simulink model "aa"  (R2025b)
settings: Solver=FixedStepAuto  StartTime=0.0  StopTime=10.0  RelTol=1e-3
libraries: androiduilib x2, dspxfrm3 x2, androidaudiovideolib x1, commchan3 x1, androidcommunicationlib x1
settings Model: Creator=chinm  LastModifiedBy=Windows
settings OptimizationCC: DefaultParameterBehavior=Inlined  EnhancedBackFolding=on  PassReuseOutputArgsAs=Individual arguments  ZeroExternalMemoryAtStartup=off  ZeroInternalMemoryAtStartup=off  MaxStackSize=64  OptimizeBlockOrder=speed  DifferentSizesBufferReuse=on  OptimizationCustomize=off  EfficientTunableParamExpr=on
settings DebuggingCC: ParameterTunabilityLossMsg=error
settings HardwareCC: ProdBitPerPointer=32.0  ProdBitPerSizeT=32.0  ProdBitPerPtrDiffT=32.0  ProdLargestAtomicInteger=Long  ProdLargestAtomicFloat=Double  ProdWordSize=32.0  ProdHWDeviceType=ARM Compatible->ARM Cortex-A (32-bit)
settings SFSimCC: MATLABDynamicMemAlloc=off
settings RTWCC: SystemTargetFile=ert.tlc  HardwareBoard=Android Device  TLCOptions="-aInlineSetEventsForThisBaseRateFcn=TLC_FALSE -aSuppressMultiTaskScheduler=TLC_FALSE  -aRateBasedStepFcn=0"  TemplateMakefile=ert_default_tmf  RTWVerbose=off  Toolchain=Android SDK/NDK Tools  GPUComputeCapability=3.5  Description=Embedded Coder
settings CodeAppCC: ForceParamTrailComments=on  IgnoreCustomStorageClasses=off  OperatorAnnotations=on  SimulinkDataObjDesc=on  SFDataObjDesc=on  InsertBlockDesc=on

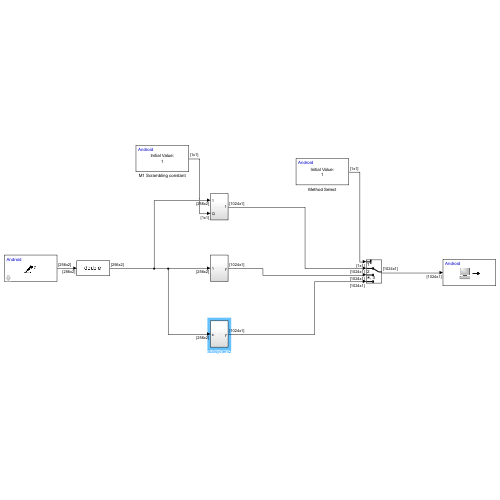
[thumbnail: Simulink's stored preview of the top-level diagram]
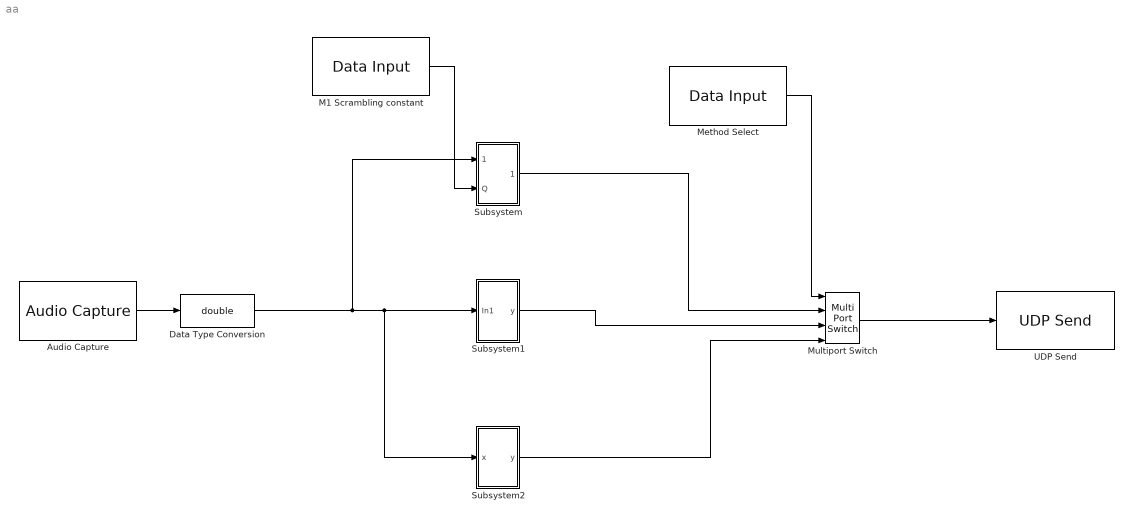
== system aa ==
  Audio Capture : androidaudiovideolib/Audio Capture  SampleFreq=8000  FrameSize=256  SampleTime=0.032  SimulateUsing=Code generation  DeviceStr=0  QueueDuration=0  BlockPlatform=Android  AudioSamplingFreq=44100
  Data Type Conversion : DataTypeConversion  OutDataTypeStr=double  SaturateOnIntegerOverflow=off  RndMeth=Floor
  M1 Scrambling constant : androiduilib/Data Input  isCharVector=off  Value=1.0  CharVector=Hello World  OutputDataType=int8  maxCharVectorSize=100  DataInputId=aa/M1_Scrambling_constant  SampleTime=1
  Method Select : androiduilib/Data Input  isCharVector=off  Value=1  CharVector=Hello World  OutputDataType=int8  maxCharVectorSize=100  DataInputId=aa/Method_Select  SampleTime=1
  Multiport Switch : MultiPortSwitch  DataPortOrder=Specify indices  DiagnosticForDefault=None  SaturateOnIntegerOverflow=off  InputSameDT=off
  Subsystem : Subsystem
  Subsystem1 : Subsystem
  Subsystem2 : Subsystem
  UDP Send : androidcommunicationlib/UDP Send  remoteURL='10.7.16.15'  remotePort=25070  localURL='0.0.0.0'  localPortSource=Automatically determine  localPort=-1  sampletime=-1  blockPlatform=Android  separateLengthPort=0
  wires:
  Subsystem2/1(y) -> Multiport Switch/4
  M1 Scrambling constant/1 -> Subsystem/2(Q)
  Method Select/1 -> Multiport Switch/1
  Subsystem/1(Out1) -> Multiport Switch/2
  Audio Capture/1 -> Data Type Conversion/1
  Subsystem1/1(y) -> Multiport Switch/3
  Multiport Switch/1 -> UDP Send/1
  Data Type Conversion/1 -> Subsystem2/1(x), Subsystem1/1(In1), Subsystem/1(In1)

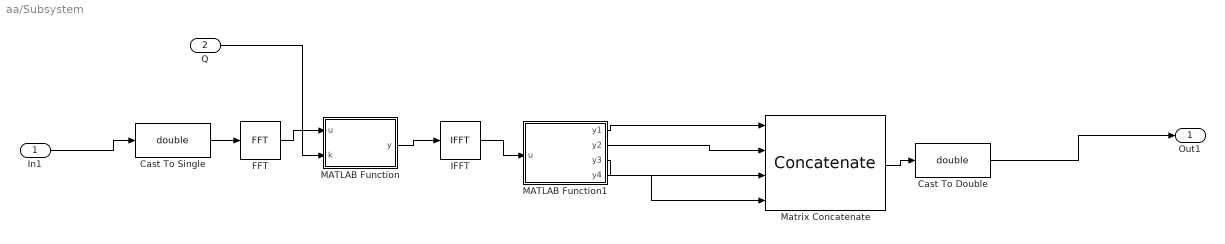
== system aa/Subsystem ==
  In1 : Inport
  Q : Inport  Port=2
  Cast To Double : DataTypeConversion  OutDataTypeStr=double  SaturateOnIntegerOverflow=off  RndMeth=Floor
  Cast To Single : DataTypeConversion  OutDataTypeStr=double  SaturateOnIntegerOverflow=off  RndMeth=Floor
  FFT : dspxfrm3/FFT  FFTImplementation=Auto  CompMethod=Table lookup  TableOpt=NEW  TableOptActive=Speed  BitRevOrder=off  Normalize=off  InheritFFTLength=on  FFTLength=64  WrapInput=on  roundingMode=Ceiling  overflowMode=off  firstCoeffDataTypeStr=Inherit: Same word length as input  firstCoeffLastDataTypeStr=Inherit: Same word length as input  outputMin=[]  outputMax=[]
  IFFT : dspxfrm3/IFFT  FFTImplementation=Auto  CompMethod=Table lookup  TableOpt=NEW  TableOptActive=Speed  BitRevOrder=off  cs_in=off  Normalize=on  InheritFFTLength=on  FFTLength=64  WrapInput=on  mode=Real  outSamplingMode=Sample based  roundingMode=Ceiling  overflowMode=off  firstCoeffDataTypeStr=Inherit: Same word length as input  firstCoeffLastDataTypeStr=Inherit: Same word length as input  outputMin=[]  outputMax=[]
  MATLAB Function : MATLAB Function  TreatAsAtomicUnit=on
  MATLAB Function1 : MATLAB Function  TreatAsAtomicUnit=on
  Matrix Concatenate : Concatenate  NumInputs=4  Mode=Multidimensional array
  Out1 : Outport
  wires:
  Cast To Double/1 -> Out1/1
  IFFT/1 -> MATLAB Function1/1(u)
  MATLAB Function1/4(y4) -> Matrix Concatenate/4
  In1/1 -> Cast To Single/1
  MATLAB Function1/2(y2) -> Matrix Concatenate/2
  Matrix Concatenate/1 -> Cast To Double/1
  Q/1 -> MATLAB Function/2(k)
  FFT/1 -> MATLAB Function/1(u)
  MATLAB Function1/3(y3) -> Matrix Concatenate/3
  MATLAB Function1/1(y1) -> Matrix Concatenate/1
  Cast To Single/1 -> FFT/1
  MATLAB Function/1(y) -> IFFT/1

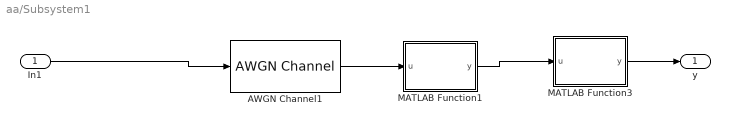
== system aa/Subsystem1 ==
  In1 : Inport  OutDataTypeStr=double
  AWGN Channel1 : commchan3/AWGN Channel  LegacyMode=on  NoiseMethod="Signal to noise ratio  (SNR)"  noiseMode="Signal to noise ratio  (SNR)"  EbNo=10  EsNo=10  SNR=10  BitsPerSymbol=1  SignalPower=1  SpecifySymbolPeriod=off  SamplesPerSymbol=1  SymbolPeriod=1  VarianceSource=Parameter  Variance=1  RandomStream=Global stream  Seed=67  SimulateUsing=Code generation
  MATLAB Function1 : MATLAB Function  TreatAsAtomicUnit=on
  MATLAB Function3 : MATLAB Function  TreatAsAtomicUnit=on
  y : Outport
  wires:
  MATLAB Function1/1(y) -> MATLAB Function3/1(u)
  AWGN Channel1/1 -> MATLAB Function1/1(u)
  In1/1 -> AWGN Channel1/1
  MATLAB Function3/1(y) -> y/1

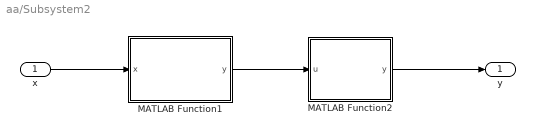
== system aa/Subsystem2 ==
  x : Inport
  MATLAB Function1 : MATLAB Function  TreatAsAtomicUnit=on
  MATLAB Function2 : MATLAB Function  TreatAsAtomicUnit=on
  y : Outport
  wires:
  x/1 -> MATLAB Function1/1(x)
  MATLAB Function1/1(y) -> MATLAB Function2/1(u)
  MATLAB Function2/1(y) -> y/1

== matlab function aa/Subsystem2/MATLAB Function2 ==
  data: u input; y output
function y = fcn(u)
    y = randn(1024,1);
    y(1:256) = u(:,1);
    y(257:512) = u(:,2);
    y(513:768) = u(:,1);
    y(769:1024) = u(:,2);
end

== matlab function aa/Subsystem1/MATLAB Function1 ==
  data: u input; y output
function y = fcn(u)
y = randn(512,1);
y(1:256) = u(:,1);
y(257:512) = u(:,2);

== matlab function aa/Subsystem/MATLAB Function ==
  data: u input; k input; y output
function y = scramble_stereo_fft(u, k)
    left_channel_fft = u(:, 1);
    right_channel_fft = u(:, 2);

    scrambled_left = scramble_channel(left_channel_fft, k);
    scrambled_right = scramble_channel(right_channel_fft, k);
    
    y = [scrambled_left, scrambled_right];
end

function scrambled_ch = scramble_channel(ch, k)
    N = length(ch);
    scrambled_ch = complex(zeros(N, 1));
    shift_amount = k*13; 
    
    for i = 1:N
        new_i = mod(i - 1 + shift_amount, N) + 1;
        scrambled_ch(new_i) = ch(i);
    end
end

== matlab function aa/Subsystem/MATLAB Function1 ==
  data: u input; y1 output; y2 output; y3 output; y4 output
function [y1,y2,y3,y4] = fcn(u)
    y1 = real(u(:,1));
    y2 = real(u(:,2));
    y3 = imag(u(:,1));
    y4 = imag(u(:,2));
end

== matlab function aa/Subsystem2/MATLAB Function1 ==
  data: x input; y output
function y = embed_watermark(x)

persistent key amp Fs
if isempty(key)
    key = 12345;
    amp = 0.05;
    Fs = 44100;
end

% --- Watermark Parameters for Audibility ---
watermark_freq = 100;  % Low-frequency tone (easy to hear)
watermark_phase = 2*pi * (key / 100000);

[N, C] = size(x);
y = zeros(N, C);
t = (0:N-1)' / Fs;

% --- Generate the Audible Sinusoidal Watermark ---
w = amp * sin(2*pi * watermark_freq * t + watermark_phase);

% --- Embed the Watermark ---
for c = 1:C
    y(:,c) = x(:,c) + w;
    y(:,c) = max(-1, min(1, y(:,c)));
end
end

== matlab function aa/Subsystem1/MATLAB Function3 ==
  data: u input; y output
function y = fcn(u)
y = randn(1024,1);
y(1:512) = u;
y(513:1024) = u;
